simulink model "FCC_replacement"  (R2018a)
settings: Solver=FixedStepDiscrete  StartTime=0.0  StopTime=10.0  FixedStep=0.001  RelTol=1e-3  EnableMultiTasking=on
undefined symbols (not defined in the file or in its folder): DiscIntNeverNeededParam
libraries: simulink x10, HeliLibrary x3
Description:
  | This model represents a flight control system for a helicopter that controls pitch attitude, roll attitude and yaw rate based on pilot inputs from the cyclic and pedals. The flight control computer also closes the loop on three hydrualic actuators and has sensor inputs from three Attitude/Heading Reference Systems.
settings Model: sldv_blockreplacement_configurable_lib=FCC_rt_lib  Creator=bpotter  LastModifiedBy=bpotter
settings DataIOCC: LimitDataPoints=on
settings OptimizationCC: BlockReduction=off  DefaultParameterBehavior=Inlined  UseDivisionForNetSlopeComputation=on  InitFltsAndDblsToZero=on  EfficientFloat2IntCast=on  EfficientMapNaN2IntZero=off  LifeSpan=inf  MaxStackSize=inf
settings DebuggingCC: SignalInfNanChecking=error  SignalRangeChecking=error  ReadBeforeWriteMsg=EnableAllAsError  WriteAfterWriteMsg=EnableAllAsError  WriteAfterReadMsg=EnableAllAsError  AlgebraicLoopMsg=error  ArtificialAlgebraicLoopMsg=error  SaveWithDisabledLinksMsg=error  SaveWithParameterizedLinksMsg=none  BlockPriorityViolationMsg=error  SolverPrmCheckMsg=error  InheritedTsInSrcMsg=error  SigSpecEnsureSampleTimeMsg=error  CheckMatrixSingularityMsg=error  IntegerOverflowMsg=error  ParameterUnderflowMsg=error  ParameterPrecisionLossMsg=error  ParameterTunabilityLossMsg=error  UnderSpecifiedDataTypeMsg=error  UnnecessaryDatatypeConvMsg=warning  VectorMatrixConversionMsg=error  UnconnectedInputMsg=error  UnconnectedOutputMsg=error  UnconnectedLineMsg=error  SFcnCompatibilityMsg=error  BusObjectLabelMismatch=error  RootOutportRequireBusObject=error  AssertControl=DisableAll  AllowSymbolicDim=off  ModelReferenceIOMsg=error  ModelReferenceIOMismatchMessage=error  UnknownTsInhSupMsg=error  ModelReferenceDataLoggingMessage=error  StateNameClashWarn=warning  StrictBusMsg=ErrorOnBusTreatedAsVector  NonBusSignalsTreatedAsBus=error  SFInvalidInputDataAccessInChartInitDiag=error  SFTransitionOutsideNaturalParentDiag=error  SFUnreachableExecutionPathDiag=error  SFUndirectedBroadcastEventsDiag=error  SFTransitionActionBeforeConditionDiag=error  SFExecutionAtInitializationDiag=none  IntegerSaturationMsg=error
settings HardwareCC: ProdBitPerPointer=32  ProdBitPerSizeT=32  ProdBitPerPtrDiffT=32  ProdLargestAtomicFloat=None  ProdEndianess=Unspecified  ProdWordSize=32  ProdHWDeviceType=32-bit Generic  TargetIntDivRoundTo=Zero
settings ModelReferenceCC: PropagateSignalLabelsOutOfModel=off
settings SFSimCC: MATLABDynamicMemAlloc=off
settings RTWCC: SystemTargetFile=ert.tlc  TemplateMakefile=ert_default_tmf  GenerateReport=on  Toolchain=LCC-win64 v2.4.1 | gmake (64-bit Windows)  IncludeHyperlinkInReport=on  LaunchReport=on  PortableWordSizes=on  GenerateTraceInfo=on  GenerateTraceReport=on  GenerateTraceReportSl=on  GenerateTraceReportSf=on  GenerateTraceReportEml=on
settings CodeAppCC: ForceParamTrailComments=on  IgnoreCustomStorageClasses=off  MangleLength=4  StateflowObjectComments=on  ReqsInCode=on
settings ERTTargetCC: TargetLangStandard=C99 (ISO)  UtilityFuncGeneration=Shared location  MultiwordLength=2048  GenerateSampleERTMain=on  IncludeMdlTerminateFcn=off  SuppressErrorStatus=on  SupportAbsoluteTime=off  SupportNonFinite=off  ParenthesesLevel=Maximum  CastingMode=Standards  GenerateSharedConstants=off  ERTCustomFileTemplate=example_file_process.tlc  PreserveExpressionOrder=on  PreserveIfCondition=on  ConvertIfToSwitch=off  SuppressUnreachableDefaultCases=off  EnableSignedLeftShifts=off  EnableSignedRightShifts=off
settings ConfigComp: CovMetricSettings=dw  CovHtmlReporting=on  CovSaveCumulativeToWorkspaceVar=on  CovSaveSingleToWorkspaceVar=on  CovExternalEMLEnable=off  CovSFcnEnable=off  PSOpenProjectManager=on  PSResultDir=CodeProver_results_$ModelName$  PSModelRefVerifDepth=All  PSAutoStubLUT=off  DVTestSuiteOptimization=CombinedObjectives (Nonlinear Extended)  DVDesignMinMaxCheck=on  DVDetectOutOfBounds=on  DVDetectFloatOverflow=off

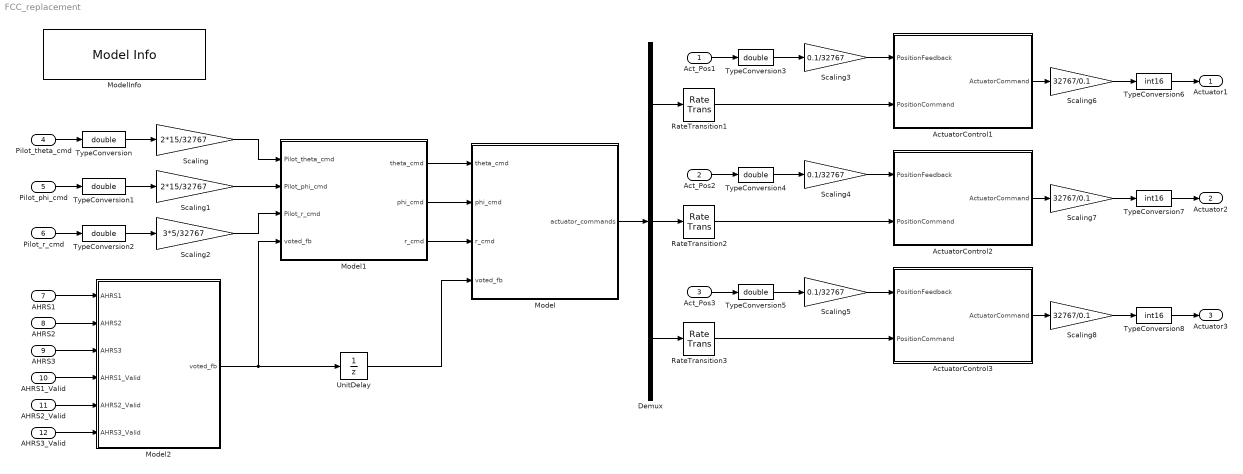
== system FCC_replacement ==
  Act_Pos1 : Inport  RequirementInfo={} %GIDa_bd07c6dd_f370_4b97_930d_e4b4981f6696  OutMin=-32768  OutMax=32767  OutDataTypeStr=int16  PortDimensions=1  SampleTime=0.001
  Act_Pos2 : Inport  RequirementInfo={} %GIDa_befe8f2a_df1a_408c_ad43_982e86d61679  Port=2  OutMin=-32768  OutMax=32767  OutDataTypeStr=int16  PortDimensions=1  SampleTime=0.001
  Act_Pos3 : Inport  RequirementInfo={} %GIDa_31a40888_6c46_41b4_95a0_85353469c339  Port=3  OutMin=-32768  OutMax=32767  OutDataTypeStr=int16  PortDimensions=1  SampleTime=0.001
  Pilot_theta_cmd : Inport  RequirementInfo={} %GIDa_db7610c8_fc0b_436a_9176_d063f912f7d4  Port=4  OutMin=-32768  OutMax=32767  OutDataTypeStr=int16  PortDimensions=1  SampleTime=0.01
  Pilot_phi_cmd : Inport  RequirementInfo={} %GIDa_c88793d4_8072_44c9_b7b8_fa9c7a9d095b  Port=5  OutMin=-32768  OutMax=32767  OutDataTypeStr=int16  PortDimensions=1  SampleTime=0.01
  Pilot_r_cmd : Inport  RequirementInfo={} %GIDa_dcbca35e_d37f_4666_ab6e_90461c32e72b  Port=6  OutMin=-32768  OutMax=32767  OutDataTypeStr=int16  PortDimensions=1  SampleTime=0.01
  AHRS1 : Inport  RequirementInfo={} %GIDa_80750aa2_e003_442f_b031_591405abb5b4  Port=7  OutMin=-180  OutMax=180  OutDataTypeStr=double  PortDimensions=5  SampleTime=0.01
  AHRS2 : Inport  RequirementInfo={} %GIDa_426ecfe9_991d_4f5f_80a1_3ebd9c43cb2d  Port=8  OutMin=-180  OutMax=180  OutDataTypeStr=double  PortDimensions=5  SampleTime=0.01
  AHRS3 : Inport  RequirementInfo={} %GIDa_78c653e8_6a57_498e_82a6_5c1330482b46  Port=9  OutMin=-180  OutMax=180  OutDataTypeStr=double  PortDimensions=5  SampleTime=0.01
  AHRS1_Valid : Inport  RequirementInfo={} %GIDa_98b30cb9_b983_4ea0_884e_7d00cc40e0ae  Port=10  OutMin=0  OutMax=1  OutDataTypeStr=boolean  PortDimensions=1  SampleTime=0.01
  AHRS2_Valid : Inport  RequirementInfo={} %GIDa_97bebaab_bb97_4960_9c93_3ab597d65b2c  Port=11  OutMin=0  OutMax=1  OutDataTypeStr=boolean  PortDimensions=1  SampleTime=0.01
  AHRS3_Valid : Inport  RequirementInfo={} %GIDa_19fd269e_922e_4b90_a0a1_f582c1a1233f  Port=12  OutMin=0  OutMax=1  OutDataTypeStr=boolean  PortDimensions=1  SampleTime=0.01
  ActuatorControl1 : Subsystem  TreatAsAtomicUnit=on  mask(Sldv ModelReference(Model name:ActuatorLoop) Replacement){ModelName=ActuatorLoop, ParameterArgumentNames=Kp,Kd,Ki, ParameterArgumentValuesAsString=0.3,0.02,0.12, SimulationMode=Normal, Kd=0.02, Ki=0.12, Kp=0.3}
      mask help: Replacement for the Model Reference block that references the model ActuatorLoop. If Model arguments are specified on the Model Reference block, then they will appear in the mask parameters.
  ActuatorControl2 : Subsystem  TreatAsAtomicUnit=on  mask(Sldv ModelReference(Model name:ActuatorLoop) Replacement){ModelName=ActuatorLoop, ParameterArgumentNames=Kp,Kd,Ki, ParameterArgumentValuesAsString=0.3,0.02,0.12, SimulationMode=Normal, Kd=0.02, Ki=0.12, Kp=0.3}
      mask help: Replacement for the Model Reference block that references the model ActuatorLoop. If Model arguments are specified on the Model Reference block, then they will appear in the mask parameters.
  ActuatorControl3 : Subsystem  TreatAsAtomicUnit=on  mask(Sldv ModelReference(Model name:ActuatorLoop) Replacement){ModelName=ActuatorLoop, ParameterArgumentNames=Kp,Kd,Ki, ParameterArgumentValuesAsString=0.3,0.02,0.12, SimulationMode=Normal, Kd=0.02, Ki=0.12, Kp=0.3}
      mask help: Replacement for the Model Reference block that references the model ActuatorLoop. If Model arguments are specified on the Model Reference block, then they will appear in the mask parameters.
  Demux : Demux  Outputs=3
  Model : Subsystem  TreatAsAtomicUnit=on  mask(Sldv ModelReference(Model name:Heli_inner_loop) Replacement){ModelName=Heli_inner_loop, ParameterArgumentNames=, ParameterArgumentValuesAsString=, SimulationMode=Normal}
      mask help: Replacement for the Model Reference block that references the model Heli_inner_loop. If Model arguments are specified on the Model Reference block, then they will appear in the mask parameters.
  Model1 : Subsystem  TreatAsAtomicUnit=on  mask(Sldv ModelReference(Model name:Heli_outer_loop) Replacement){ModelName=Heli_outer_loop, ParameterArgumentNames=, ParameterArgumentValuesAsString=, SimulationMode=Normal}
      mask help: Replacement for the Model Reference block that references the model Heli_outer_loop. If Model arguments are specified on the Model Reference block, then they will appear in the mask parameters.
  Model2 : Subsystem  TreatAsAtomicUnit=on  mask(Sldv ModelReference(Model name:AHRS_voter) Replacement){ModelName=AHRS_voter, ParameterArgumentNames=, ParameterArgumentValuesAsString=, SimulationMode=Normal}
      mask help: Replacement for the Model Reference block that references the model AHRS_voter. If Model arguments are specified on the Model Reference block, then they will appear in the mask parameters.
  ModelInfo : simulink/Model-Wide Utilities/Model Info  Frame=on  DisplayStringWithTags=|  HorizontalTextAlignment=Center  LeftAlignmentValue=0.5
      | Model Name: %<ModelName>
      | Model Version: %<ModelVersion>
      | Last Modified: %<LastModificationDate>
      | 
      | Copyright 2016 The MathWorks, Inc.
  RateTransition1 : RateTransition  OutPortSampleTime=0.001
  RateTransition2 : RateTransition  OutPortSampleTime=0.001
  RateTransition3 : RateTransition  OutPortSampleTime=0.001
  Scaling : Gain  RequirementInfo={} %GIDa_1ef55a73_43a4_45d8_95fb_e076cecdcdfb  Gain=2*15/32767
  Scaling1 : Gain  RequirementInfo={} %GIDa_7c0c4402_eed7_48e8_afe7_4e3c25c20a7a  Gain=2*15/32767
  Scaling2 : Gain  RequirementInfo={} %GIDa_c573d4b7_5d38_46e9_91de_b74deab4371c  Gain=3*5/32767
  Scaling3 : Gain  RequirementInfo={} %GIDa_7165c314_723d_4c07_8145_b8a5caf68d15  Gain=0.1/32767
  Scaling4 : Gain  RequirementInfo={} %GIDa_e7d939dc_4756_4c7f_b09b_37bf3b41d91a  Gain=0.1/32767
  Scaling5 : Gain  RequirementInfo={} %GIDa_feb82ae6_ad6e_4307_be71_c8336adce306  Gain=0.1/32767
  Scaling6 : Gain  RequirementInfo={} %GIDa_7472457d_0776_496d_982d_888a9d0ccd31  Gain=32767/0.1  SaturateOnIntegerOverflow=on  OutDataTypeStr=Inherit: Same as input
  Scaling7 : Gain  RequirementInfo={} %GIDa_27270bf9_988e_4404_bcbc_b8b952500a10  Gain=32767/0.1  SaturateOnIntegerOverflow=on  OutDataTypeStr=Inherit: Same as input
  Scaling8 : Gain  RequirementInfo={} %GIDa_610bafad_081e_4b34_b128_56987096ac68  Gain=32767/0.1  SaturateOnIntegerOverflow=on  OutDataTypeStr=Inherit: Same as input
  TypeConversion : DataTypeConversion  RequirementInfo={} %GIDa_507dfc48_2783_4f54_bcc8_b8696a72db7e  OutDataTypeStr=double
  TypeConversion1 : DataTypeConversion  RequirementInfo={} %GIDa_a28ee961_0826_464b_952a_7525a850e69d  OutDataTypeStr=double
  TypeConversion2 : DataTypeConversion  RequirementInfo={} %GIDa_fd029ccd_092a_44ae_ba63_7ba73a38dd29  OutDataTypeStr=double
  TypeConversion3 : DataTypeConversion  RequirementInfo={} %GIDa_1949c14f_f47a_4a2c_b83b_c5a889847ffe  OutDataTypeStr=double
  TypeConversion4 : DataTypeConversion  RequirementInfo={} %GIDa_29dd9675_a919_4bb5_a5f8_82f3a5941f34  OutDataTypeStr=double
  TypeConversion5 : DataTypeConversion  RequirementInfo={} %GIDa_0de29fa2_9bc9_4717_a2b2_9bc25147b395  OutDataTypeStr=double
  TypeConversion6 : DataTypeConversion  RequirementInfo={} %GIDa_6ab4c5ff_fe2f_4ca3_924f_fd1b53f5822d  OutDataTypeStr=int16
  TypeConversion7 : DataTypeConversion  RequirementInfo={} %GIDa_fe351f61_f1d0_4404_aa3c_5114a8d4af07  OutDataTypeStr=int16
  TypeConversion8 : DataTypeConversion  RequirementInfo={} %GIDa_5d4fc6d9_c4e4_4413_b6aa_2af104ad7bd2  OutDataTypeStr=int16
  UnitDelay : UnitDelay  SampleTime=-1
  Actuator1 : Outport  RequirementInfo={} %GIDa_0e27a381_736b_4604_a443_1ce3b6bc89bb
  Actuator2 : Outport  RequirementInfo={} %GIDa_ad165c3e_4ab6_4671_aa0b_225d448592bb  Port=2
  Actuator3 : Outport  RequirementInfo={} %GIDa_f2f33165_edb5_46cb_9250_52960ae67539  Port=3
  wires:
  ActuatorControl1/1(ActuatorCommand) -> Scaling6/1
  ActuatorControl2/1(ActuatorCommand) -> Scaling7/1
  ActuatorControl3/1(ActuatorCommand) -> Scaling8/1
  RateTransition1/1 -> ActuatorControl1/2(PositionCommand)
  RateTransition2/1 -> ActuatorControl2/2(PositionCommand)
  RateTransition3/1 -> ActuatorControl3/2(PositionCommand)
  AHRS2/1 -> Model2/2(AHRS2)
  AHRS3/1 -> Model2/3(AHRS3)
  Demux/1 -> RateTransition1/1
  Demux/2 -> RateTransition2/1
  Demux/3 -> RateTransition3/1
  Model/1(actuator_commands) -> Demux/1
  Model1/1(theta_cmd) -> Model/1(theta_cmd)
  Model1/2(phi_cmd) -> Model/2(phi_cmd)
  Model1/3(r_cmd) -> Model/3(r_cmd)
  AHRS1/1 -> Model2/1(AHRS1)
  Model2/1(voted_fb) -> Model1/4(voted_fb), UnitDelay/1
  AHRS1_Valid/1 -> Model2/4(AHRS1_Valid)
  AHRS2_Valid/1 -> Model2/5(AHRS2_Valid)
  AHRS3_Valid/1 -> Model2/6(AHRS3_Valid)
  TypeConversion/1 -> Scaling/1
  Pilot_theta_cmd/1 -> TypeConversion/1
  Scaling/1 -> Model1/1(Pilot_theta_cmd)
  TypeConversion1/1 -> Scaling1/1
  Pilot_phi_cmd/1 -> TypeConversion1/1
  Scaling1/1 -> Model1/2(Pilot_phi_cmd)
  Pilot_r_cmd/1 -> TypeConversion2/1
  TypeConversion2/1 -> Scaling2/1
  Scaling2/1 -> Model1/3(Pilot_r_cmd)
  TypeConversion3/1 -> Scaling3/1
  Act_Pos1/1 -> TypeConversion3/1
  Scaling3/1 -> ActuatorControl1/1(PositionFeedback)
  TypeConversion4/1 -> Scaling4/1
  TypeConversion5/1 -> Scaling5/1
  Act_Pos2/1 -> TypeConversion4/1
  Scaling4/1 -> ActuatorControl2/1(PositionFeedback)
  Act_Pos3/1 -> TypeConversion5/1
  Scaling5/1 -> ActuatorControl3/1(PositionFeedback)
  Scaling6/1 -> TypeConversion6/1
  Scaling7/1 -> TypeConversion7/1
  Scaling8/1 -> TypeConversion8/1
  TypeConversion6/1 -> Actuator1/1
  TypeConversion7/1 -> Actuator2/1
  TypeConversion8/1 -> Actuator3/1
  UnitDelay/1 -> Model/4(voted_fb)

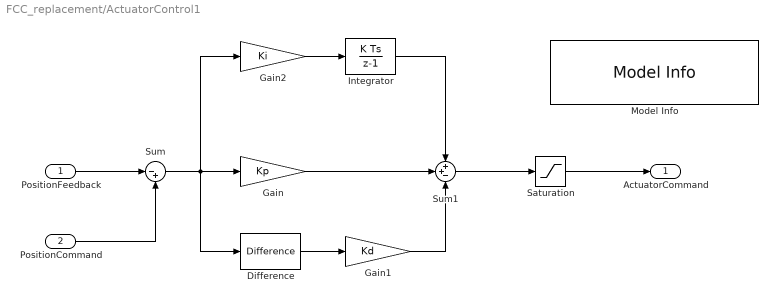
== system FCC_replacement/ActuatorControl1 ==
  PositionFeedback : Inport  OutMin=-0.1  OutMax=0.1  OutDataTypeStr=double  PortDimensions=1  SampleTime=[0.001,0]
  PositionCommand : Inport  Port=2  OutMin=-0.1  OutMax=0.1  OutDataTypeStr=double  PortDimensions=1  SampleTime=[0.001,0]
  Difference : simulink/Discrete/Difference  ICPrevInput=0.0  OutMin=[]  OutMax=[]  OutDataType=fixdt(1, 16)  OutScaling=2^-10  DoSatur=off
  Gain : Gain  Gain=Kp
  Gain1 : Gain  Gain=Kd
  Gain2 : Gain  Gain=Ki
  Integrator : DiscreteIntegrator  SampleTime=-1  LimitOutput=on  UpperSaturationLimit=0.1  LowerSaturationLimit=-0.1  ICPrevOutput=DiscIntNeverNeededParam  ICPrevScaledInput=DiscIntNeverNeededParam
      settings: AttributesFormatString="%<LowerSaturationLimit> to  %<UpperSaturationLimit>"
  Model Info : simulink/Model-Wide Utilities/Model Info  Frame=on  DisplayStringWithTags=|  HorizontalTextAlignment=Center  LeftAlignmentValue=0.5
      | Model Name: %<ModelName>
      | Model Version: %<ModelVersion>
      | Last Modified: %<LastModificationDate>
      | 
      | Copyright 2016 The MathWorks, Inc.
  Saturation : Saturate  UpperLimit=0.3  LowerLimit=-0.3
      settings: AttributesFormatString=%<LowerLimit> to %<UpperLimit>
  Sum : Sum  Inputs=|-+
  Sum1 : Sum  Inputs=++-
  ActuatorCommand : Outport  OutDataTypeStr=double  PortDimensions=1  SampleTime=[0.001,0]
  wires:
  Saturation/1 -> ActuatorCommand/1
  Gain2/1 -> Integrator/1
  Gain1/1 -> Sum1/3
  Difference/1 -> Gain1/1
  Integrator/1 -> Sum1/1
  Sum1/1 -> Saturation/1
  Gain/1 -> Sum1/2
  Sum/1 -> Difference/1, Gain2/1, Gain/1
  PositionCommand/1 -> Sum/2
  PositionFeedback/1 -> Sum/1

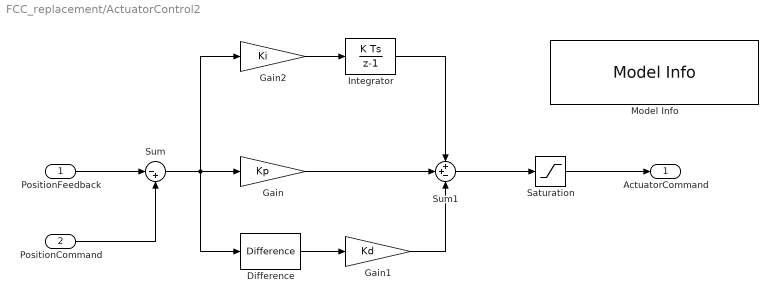
== system FCC_replacement/ActuatorControl2 ==
  PositionFeedback : Inport  OutMin=-0.1  OutMax=0.1  OutDataTypeStr=double  PortDimensions=1  SampleTime=[0.001,0]
  PositionCommand : Inport  Port=2  OutMin=-0.1  OutMax=0.1  OutDataTypeStr=double  PortDimensions=1  SampleTime=[0.001,0]
  Difference : simulink/Discrete/Difference  ICPrevInput=0.0  OutMin=[]  OutMax=[]  OutDataType=fixdt(1, 16)  OutScaling=2^-10  DoSatur=off
  Gain : Gain  Gain=Kp
  Gain1 : Gain  Gain=Kd
  Gain2 : Gain  Gain=Ki
  Integrator : DiscreteIntegrator  SampleTime=-1  LimitOutput=on  UpperSaturationLimit=0.1  LowerSaturationLimit=-0.1  ICPrevOutput=DiscIntNeverNeededParam  ICPrevScaledInput=DiscIntNeverNeededParam
      settings: AttributesFormatString="%<LowerSaturationLimit> to  %<UpperSaturationLimit>"
  Model Info : simulink/Model-Wide Utilities/Model Info  Frame=on  DisplayStringWithTags=|  HorizontalTextAlignment=Center  LeftAlignmentValue=0.5
      | Model Name: %<ModelName>
      | Model Version: %<ModelVersion>
      | Last Modified: %<LastModificationDate>
      | 
      | Copyright 2016 The MathWorks, Inc.
  Saturation : Saturate  UpperLimit=0.3  LowerLimit=-0.3
      settings: AttributesFormatString=%<LowerLimit> to %<UpperLimit>
  Sum : Sum  Inputs=|-+
  Sum1 : Sum  Inputs=++-
  ActuatorCommand : Outport  OutDataTypeStr=double  PortDimensions=1  SampleTime=[0.001,0]
  wires:
  Saturation/1 -> ActuatorCommand/1
  Gain2/1 -> Integrator/1
  Gain1/1 -> Sum1/3
  Difference/1 -> Gain1/1
  Integrator/1 -> Sum1/1
  Sum1/1 -> Saturation/1
  Gain/1 -> Sum1/2
  Sum/1 -> Difference/1, Gain2/1, Gain/1
  PositionCommand/1 -> Sum/2
  PositionFeedback/1 -> Sum/1

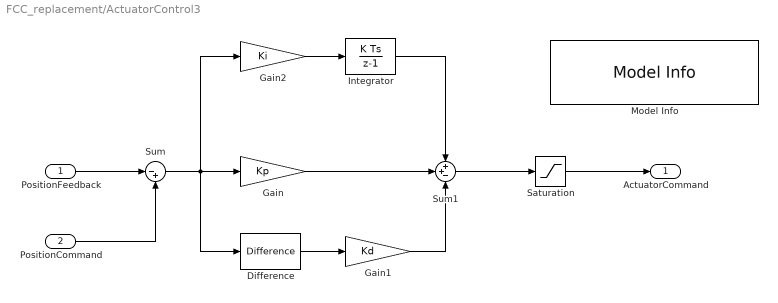
== system FCC_replacement/ActuatorControl3 ==
  PositionFeedback : Inport  OutMin=-0.1  OutMax=0.1  OutDataTypeStr=double  PortDimensions=1  SampleTime=[0.001,0]
  PositionCommand : Inport  Port=2  OutMin=-0.1  OutMax=0.1  OutDataTypeStr=double  PortDimensions=1  SampleTime=[0.001,0]
  Difference : simulink/Discrete/Difference  ICPrevInput=0.0  OutMin=[]  OutMax=[]  OutDataType=fixdt(1, 16)  OutScaling=2^-10  DoSatur=off
  Gain : Gain  Gain=Kp
  Gain1 : Gain  Gain=Kd
  Gain2 : Gain  Gain=Ki
  Integrator : DiscreteIntegrator  SampleTime=-1  LimitOutput=on  UpperSaturationLimit=0.1  LowerSaturationLimit=-0.1  ICPrevOutput=DiscIntNeverNeededParam  ICPrevScaledInput=DiscIntNeverNeededParam
      settings: AttributesFormatString="%<LowerSaturationLimit> to  %<UpperSaturationLimit>"
  Model Info : simulink/Model-Wide Utilities/Model Info  Frame=on  DisplayStringWithTags=|  HorizontalTextAlignment=Center  LeftAlignmentValue=0.5
      | Model Name: %<ModelName>
      | Model Version: %<ModelVersion>
      | Last Modified: %<LastModificationDate>
      | 
      | Copyright 2016 The MathWorks, Inc.
  Saturation : Saturate  UpperLimit=0.3  LowerLimit=-0.3
      settings: AttributesFormatString=%<LowerLimit> to %<UpperLimit>
  Sum : Sum  Inputs=|-+
  Sum1 : Sum  Inputs=++-
  ActuatorCommand : Outport  OutDataTypeStr=double  PortDimensions=1  SampleTime=[0.001,0]
  wires:
  Saturation/1 -> ActuatorCommand/1
  Gain2/1 -> Integrator/1
  Gain1/1 -> Sum1/3
  Difference/1 -> Gain1/1
  Integrator/1 -> Sum1/1
  Sum1/1 -> Saturation/1
  Gain/1 -> Sum1/2
  Sum/1 -> Difference/1, Gain2/1, Gain/1
  PositionCommand/1 -> Sum/2
  PositionFeedback/1 -> Sum/1

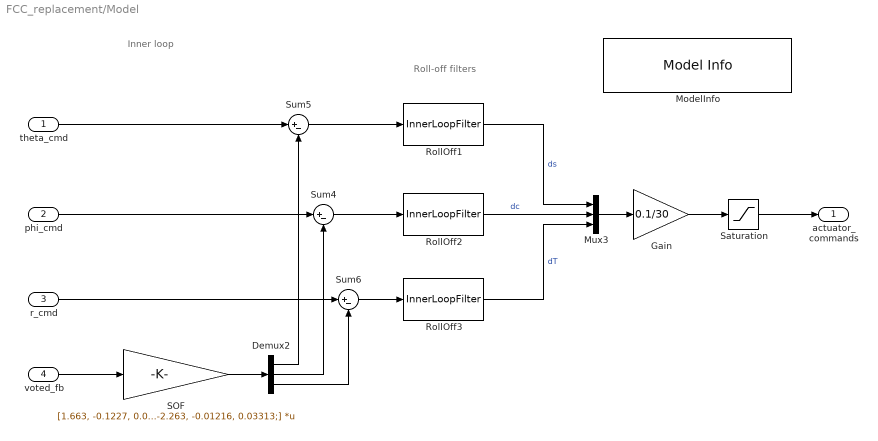
== system FCC_replacement/Model ==
  note: Inner loop
  note: Roll-off filters
  theta_cmd : Inport  OutMin=-30  OutMax=30  OutDataTypeStr=double  PortDimensions=1  SampleTime=[0.01,0]
  phi_cmd : Inport  Port=2  OutMin=-30  OutMax=30  OutDataTypeStr=double  PortDimensions=1  SampleTime=[0.01,0]
  r_cmd : Inport  Port=3  OutMin=-30  OutMax=30  OutDataTypeStr=double  PortDimensions=1  SampleTime=[0.01,0]
  voted_fb : Inport  Port=4  OutMin=-180  OutMax=180  OutDataTypeStr=double  PortDimensions=5  SampleTime=[0.01,0]
  Demux2 : Demux  Outputs=3
  Gain : Gain  Gain=0.1/30
  ModelInfo : simulink/Model-Wide Utilities/Model Info  Frame=on  DisplayStringWithTags=|  HorizontalTextAlignment=Center  LeftAlignmentValue=0.5
      | Model Name: %<ModelName>
      | Model Version: %<ModelVersion>
      | Last Modified: %<LastModificationDate>
      | 
      | Copyright 2016 The MathWorks, Inc.
  Mux3 : Mux  Inputs=3
  RollOff1 : HeliLibrary/InnerLoopFilter  Tag=FilterWizardSubSystem  SystemSampleTime=-1
      settings: AttributesFormatString=@100Hz
  RollOff2 : HeliLibrary/InnerLoopFilter  Tag=FilterWizardSubSystem  SystemSampleTime=-1
      settings: AttributesFormatString=@100Hz
  RollOff3 : HeliLibrary/InnerLoopFilter  Tag=FilterWizardSubSystem  SystemSampleTime=-1
      settings: AttributesFormatString=@100Hz
  SOF : Gain  Gain=[1.663, -0.1227, 0.09323, 0.6106, -0.0001622; -0.2907, -1.427, 0.02917, -0.07969, -0.1099; -0.002587, 0.0138, -2.263, -0.01216, 0.03313;]  Multiplication=Matrix(K*u) (u vector)
  Saturation : Saturate  UpperLimit=0.1  LowerLimit=-0.1
  Sum4 : Sum  Inputs=|+-
  Sum5 : Sum  Inputs=|+-
  Sum6 : Sum  Inputs=|+-
  actuator_commands : Outport  OutDataTypeStr=double  PortDimensions=3  SampleTime=[0.01,0]
  wires:
  Saturation/1 -> actuator_commands/1
  Gain/1 -> Saturation/1
  voted_fb/1 -> SOF/1
  Demux2/3 -> Sum6/2
  Demux2/2 -> Sum4/2
  Demux2/1 -> Sum5/2
  Sum6/1 -> RollOff3/1
  r_cmd/1 -> Sum6/1
  phi_cmd/1 -> Sum4/1
  SOF/1 -> Demux2/1
  Sum5/1 -> RollOff1/1
  theta_cmd/1 -> Sum5/1
  RollOff1/1 -> Mux3/1  "ds"
  RollOff2/1 -> Mux3/2  "dc"
  RollOff3/1 -> Mux3/3  "dT"
  Sum4/1 -> RollOff2/1
  Mux3/1 -> Gain/1

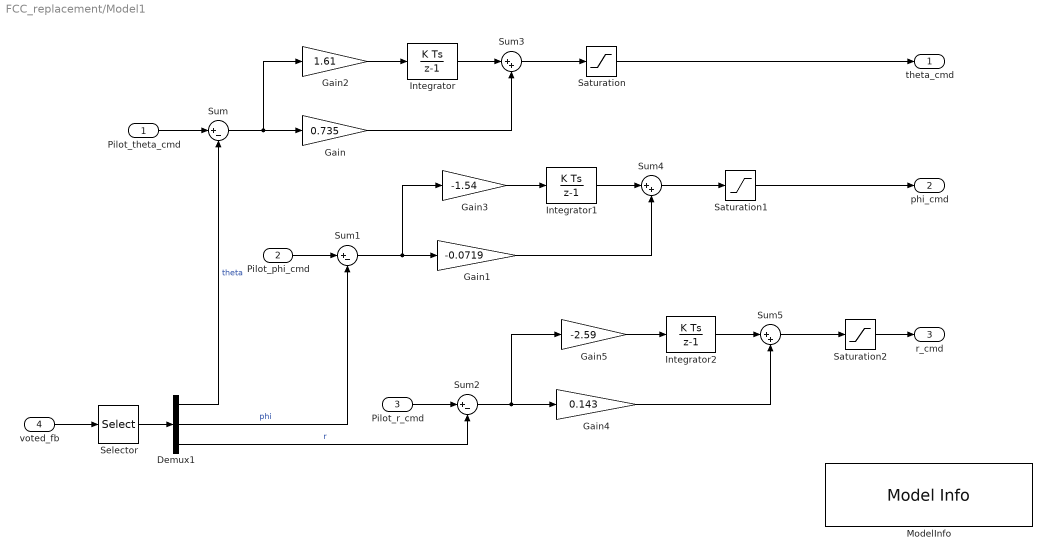
== system FCC_replacement/Model1 ==
  Pilot_theta_cmd : Inport  OutMin=-30  OutMax=30  OutDataTypeStr=double  PortDimensions=1  SampleTime=[0.01,0]
  Pilot_phi_cmd : Inport  Port=2  OutMin=-30  OutMax=30  OutDataTypeStr=double  PortDimensions=1  SampleTime=[0.01,0]
  Pilot_r_cmd : Inport  Port=3  OutMin=-15  OutMax=15  OutDataTypeStr=double  PortDimensions=1  SampleTime=[0.01,0]
  voted_fb : Inport  Port=4  OutMin=-180  OutMax=180  OutDataTypeStr=double  PortDimensions=5  SampleTime=[0.01,0]
  Demux1 : Demux  Outputs=3
  Gain : Gain  Gain=0.735
  Gain1 : Gain  Gain=-0.0719
  Gain2 : Gain  Gain=1.61
  Gain3 : Gain  Gain=-1.54
  Gain4 : Gain  Gain=0.143
  Gain5 : Gain  Gain=-2.59
  Integrator : DiscreteIntegrator  SampleTime=-1  LimitOutput=on  UpperSaturationLimit=10  LowerSaturationLimit=-10  ICPrevOutput=DiscIntNeverNeededParam  ICPrevScaledInput=DiscIntNeverNeededParam
      settings: AttributesFormatString="%<LowerSaturationLimit> to  %<UpperSaturationLimit>"
  Integrator1 : DiscreteIntegrator  SampleTime=-1  LimitOutput=on  UpperSaturationLimit=10  LowerSaturationLimit=-10  ICPrevOutput=DiscIntNeverNeededParam  ICPrevScaledInput=DiscIntNeverNeededParam
      settings: AttributesFormatString="%<LowerSaturationLimit> to  %<UpperSaturationLimit>"
  Integrator2 : DiscreteIntegrator  SampleTime=-1  LimitOutput=on  UpperSaturationLimit=10  LowerSaturationLimit=-10  ICPrevOutput=DiscIntNeverNeededParam  ICPrevScaledInput=DiscIntNeverNeededParam
      settings: AttributesFormatString="%<LowerSaturationLimit> to  %<UpperSaturationLimit>"
  ModelInfo : simulink/Model-Wide Utilities/Model Info  Frame=on  DisplayStringWithTags=|  HorizontalTextAlignment=Center  LeftAlignmentValue=0.5
      | Model Name: %<ModelName>
      | Model Version: %<ModelVersion>
      | Last Modified: %<LastModificationDate>
      | 
      | Copyright 2016 The MathWorks, Inc.
  Saturation : Saturate  UpperLimit=30  LowerLimit=-30
      settings: AttributesFormatString=%<LowerLimit> to %<UpperLimit>
  Saturation1 : Saturate  UpperLimit=30  LowerLimit=-30
      settings: AttributesFormatString=%<LowerLimit> to %<UpperLimit>
  Saturation2 : Saturate  UpperLimit=30  LowerLimit=-30
      settings: AttributesFormatString=%<LowerLimit> to %<UpperLimit>
  Selector : Selector  InputPortWidth=5  IndexOptions=Index vector (dialog)  Indices=[1 2 3]  OutputSizes=1
  Sum : Sum  Inputs=|+-  InputSameDT=on  OutDataTypeStr=Inherit: Same as first input
  Sum1 : Sum  Inputs=|+-  InputSameDT=on  OutDataTypeStr=Inherit: Same as first input
  Sum2 : Sum  Inputs=|+-  InputSameDT=on  OutDataTypeStr=Inherit: Same as first input
  Sum3 : Sum  Inputs=|++
  Sum4 : Sum  Inputs=|++
  Sum5 : Sum  Inputs=|++
  theta_cmd : Outport  OutDataTypeStr=double  PortDimensions=1  SampleTime=[0.01,0]
  phi_cmd : Outport  Port=2  OutDataTypeStr=double  PortDimensions=1  SampleTime=[0.01,0]
  r_cmd : Outport  Port=3  OutDataTypeStr=double  PortDimensions=1  SampleTime=[0.01,0]
  wires:
  Saturation2/1 -> r_cmd/1
  Sum2/1 -> Gain5/1, Gain4/1
  Gain5/1 -> Integrator2/1
  Integrator2/1 -> Sum5/1
  Sum5/1 -> Saturation2/1
  Gain4/1 -> Sum5/2
  Saturation1/1 -> phi_cmd/1
  Gain3/1 -> Integrator1/1
  Integrator1/1 -> Sum4/1
  Sum4/1 -> Saturation1/1
  Gain1/1 -> Sum4/2
  Sum1/1 -> Gain3/1, Gain1/1
  Saturation/1 -> theta_cmd/1
  Gain2/1 -> Integrator/1
  Integrator/1 -> Sum3/1
  Sum3/1 -> Saturation/1
  Gain/1 -> Sum3/2
  Sum/1 -> Gain/1, Gain2/1
  Pilot_r_cmd/1 -> Sum2/1
  Pilot_phi_cmd/1 -> Sum1/1
  Pilot_theta_cmd/1 -> Sum/1
  voted_fb/1 -> Selector/1
  Demux1/3 -> Sum2/2  "r"
  Demux1/2 -> Sum1/2  "phi"
  Demux1/1 -> Sum/2  "theta"
  Selector/1 -> Demux1/1

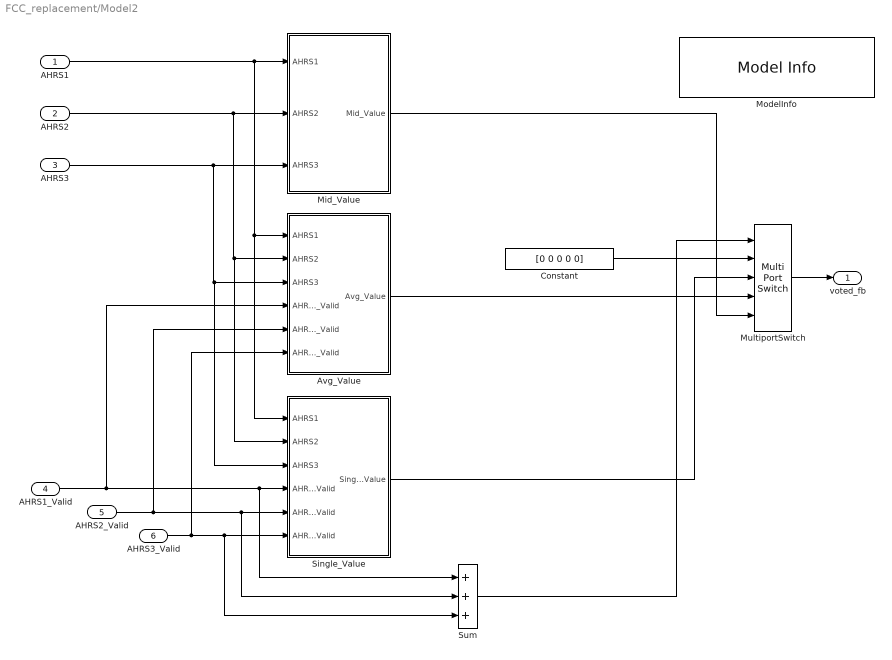
== system FCC_replacement/Model2 ==
  AHRS1 : Inport  OutMin=-180  OutMax=180  OutDataTypeStr=double  PortDimensions=5  SampleTime=[0.01,0]
  AHRS2 : Inport  Port=2  OutMin=-180  OutMax=180  OutDataTypeStr=double  PortDimensions=5  SampleTime=[0.01,0]
  AHRS3 : Inport  Port=3  OutMin=-180  OutMax=180  OutDataTypeStr=double  PortDimensions=5  SampleTime=[0.01,0]
  AHRS1_Valid : Inport  Port=4  OutMin=0  OutMax=1  OutDataTypeStr=boolean  PortDimensions=1  SampleTime=[0.01,0]
  AHRS2_Valid : Inport  Port=5  OutMin=0  OutMax=1  OutDataTypeStr=boolean  PortDimensions=1  SampleTime=[0.01,0]
  AHRS3_Valid : Inport  Port=6  OutMin=0  OutMax=1  OutDataTypeStr=boolean  PortDimensions=1  SampleTime=[0.01,0]
  Avg_Value : Subsystem  TreatAsAtomicUnit=on
      settings: RTWSystemCode=Inline
  Constant : Constant  Value=[0 0 0 0 0]
  Mid_Value : Subsystem  TreatAsAtomicUnit=on
      settings: RTWSystemCode=Inline
  ModelInfo : simulink/Model-Wide Utilities/Model Info  Frame=on  DisplayStringWithTags=|  HorizontalTextAlignment=Center  LeftAlignmentValue=0.5
      | Model Name: %<ModelName>
      | Model Version: %<ModelVersion>
      | Last Modified: %<LastModificationDate>
      | 
      | Copyright 2016 The MathWorks, Inc.
  MultiportSwitch : MultiPortSwitch  DataPortOrder=Zero-based contiguous  Inputs=4  DiagnosticForDefault=None  zeroidx=on
  Single_Value : Subsystem  TreatAsAtomicUnit=on
      settings: RTWSystemCode=Inline
  Sum : Sum  Inputs=+++  OutDataTypeStr=uint32
  voted_fb : Outport  OutDataTypeStr=double  PortDimensions=5  SampleTime=[0.01,0]
  wires:
  Constant/1 -> MultiportSwitch/2
  Single_Value/1(Single_Value) -> MultiportSwitch/3
  Avg_Value/1(Avg_Value) -> MultiportSwitch/4
  Mid_Value/1(Mid_Value) -> MultiportSwitch/5
  Sum/1 -> MultiportSwitch/1
  MultiportSwitch/1 -> voted_fb/1
  AHRS3_Valid/1 -> Sum/3, Single_Value/6(AHRS3_Valid), Avg_Value/6(AHRS3_Valid)
  AHRS2_Valid/1 -> Sum/2, Single_Value/5(AHRS2_Valid), Avg_Value/5(AHRS2_Valid)
  AHRS1_Valid/1 -> Sum/1, Single_Value/4(AHRS1_Valid), Avg_Value/4(AHRS1_Valid)
  AHRS3/1 -> Single_Value/3(AHRS3), Avg_Value/3(AHRS3), Mid_Value/3(AHRS3)
  AHRS2/1 -> Single_Value/2(AHRS2), Avg_Value/2(AHRS2), Mid_Value/2(AHRS2)
  AHRS1/1 -> Single_Value/1(AHRS1), Avg_Value/1(AHRS1), Mid_Value/1(AHRS1)

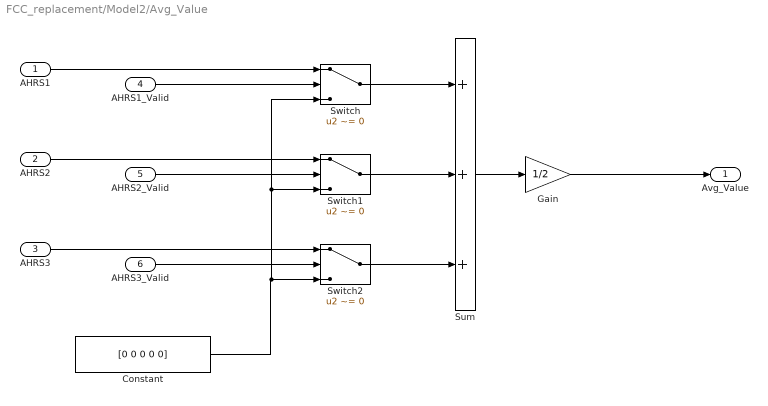
== system FCC_replacement/Model2/Avg_Value ==
  AHRS1 : Inport
  AHRS2 : Inport  Port=2
  AHRS3 : Inport  Port=3
  AHRS1_Valid : Inport  Port=4  OutDataTypeStr=boolean  PortDimensions=1
  AHRS2_Valid : Inport  Port=5  OutDataTypeStr=boolean  PortDimensions=1
  AHRS3_Valid : Inport  Port=6  OutDataTypeStr=boolean  PortDimensions=1
  Constant : Constant  Value=[0 0 0 0 0]
  Gain : Gain  Gain=1/2
  Sum : Sum  Inputs=+++
  Switch : Switch  Criteria=u2 ~= 0
  Switch1 : Switch  Criteria=u2 ~= 0
  Switch2 : Switch  Criteria=u2 ~= 0
  Avg_Value : Outport
  wires:
  Gain/1 -> Avg_Value/1
  Sum/1 -> Gain/1
  AHRS1_Valid/1 -> Switch/2
  AHRS1/1 -> Switch/1
  Switch/1 -> Sum/1
  Switch1/1 -> Sum/2
  Switch2/1 -> Sum/3
  AHRS2_Valid/1 -> Switch1/2
  AHRS3_Valid/1 -> Switch2/2
  AHRS2/1 -> Switch1/1
  AHRS3/1 -> Switch2/1
  Constant/1 -> Switch/3, Switch1/3, Switch2/3

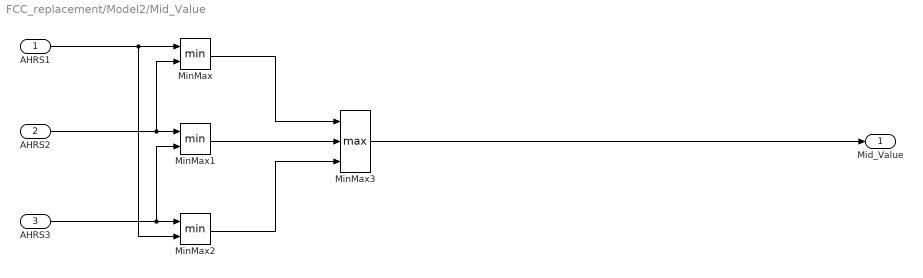
== system FCC_replacement/Model2/Mid_Value ==
  AHRS1 : Inport
  AHRS2 : Inport  Port=2
  AHRS3 : Inport  Port=3
  MinMax : MinMax  Inputs=2
  MinMax1 : MinMax  Inputs=2
  MinMax2 : MinMax  Inputs=2
  MinMax3 : MinMax  Function=max  Inputs=3
  Mid_Value : Outport
  wires:
  AHRS1/1 -> MinMax2/2, MinMax/1
  AHRS3/1 -> MinMax1/2, MinMax2/1
  AHRS2/1 -> MinMax/2, MinMax1/1
  MinMax1/1 -> MinMax3/2
  MinMax/1 -> MinMax3/1
  MinMax2/1 -> MinMax3/3
  MinMax3/1 -> Mid_Value/1

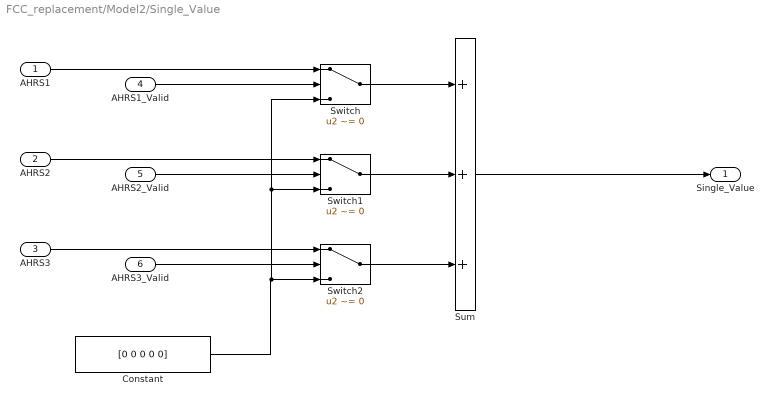
== system FCC_replacement/Model2/Single_Value ==
  AHRS1 : Inport
  AHRS2 : Inport  Port=2
  AHRS3 : Inport  Port=3
  AHRS1_Valid : Inport  Port=4  OutDataTypeStr=boolean  PortDimensions=1
  AHRS2_Valid : Inport  Port=5  OutDataTypeStr=boolean  PortDimensions=1
  AHRS3_Valid : Inport  Port=6  OutDataTypeStr=boolean  PortDimensions=1
  Constant : Constant  Value=[0 0 0 0 0]
  Sum : Sum  Inputs=+++
  Switch : Switch  Criteria=u2 ~= 0
  Switch1 : Switch  Criteria=u2 ~= 0
  Switch2 : Switch  Criteria=u2 ~= 0
  Single_Value : Outport
  wires:
  Constant/1 -> Switch2/3, Switch1/3, Switch/3
  AHRS3/1 -> Switch2/1
  AHRS2/1 -> Switch1/1
  AHRS3_Valid/1 -> Switch2/2
  AHRS2_Valid/1 -> Switch1/2
  Switch2/1 -> Sum/3
  Switch1/1 -> Sum/2
  Switch/1 -> Sum/1
  AHRS1/1 -> Switch/1
  AHRS1_Valid/1 -> Switch/2
  Sum/1 -> Single_Value/1
